simulink model "AVR"  (Simulink 7.2)
settings: Solver=ode45  StartTime=0.0  StopTime=10.0  RelTol=1e-3
libraries: simulink_extras x2
settings Model: Creator=Administrator  LastModifiedBy=huangs

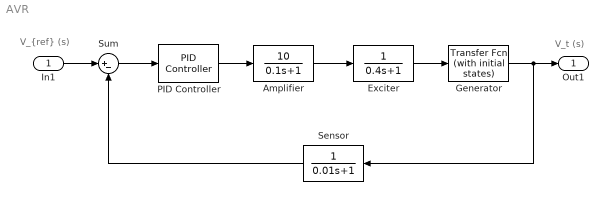
== system AVR ==
  note: V_t (s)
  note: V_{ref} (s)
  In1 : Inport  OutDataType=sfix(16)  OutScaling=2^0
  Amplifier : TransferFcn  Numerator=[10]  Denominator=[0.1 1]
  Exciter : TransferFcn  Denominator=[0.4 1]
  Generator : simulink_extras/Additional Linear/Transfer Fcn (with initial states)  SystemSampleTime=-1  N=[1]  D="[1  1]"  X0=.5
  PID Controller : simulink_extras/Additional Linear/PID Controller  SystemSampleTime=-1  P=1  I=1  D=0
  Sensor : TransferFcn  Orientation=left  Denominator=[0.01 1]
  Sum : Sum  Inputs=|+-  OutDataType=sfix(16)  OutScaling=2^0
  Out1 : Outport  OutDataType=sfix(16)  OutScaling=2^0
  wires:
  Exciter/1 -> Generator/1
  Amplifier/1 -> Exciter/1
  PID Controller/1 -> Amplifier/1
  Sensor/1 -> Sum/2
  Sum/1 -> PID Controller/1
  In1/1 -> Sum/1
  Generator/1 -> Sensor/1, Out1/1
